simulink subsystem "snake_main_model"  (R2022a)
settings: Solver=VariableStepAuto  StartTime=0.0  StopTime=10.0  RelTol=1e-3
settings Model: DefaultTestHarness=snake_main_model_harness  Creator=andre  LastModifiedBy=andre

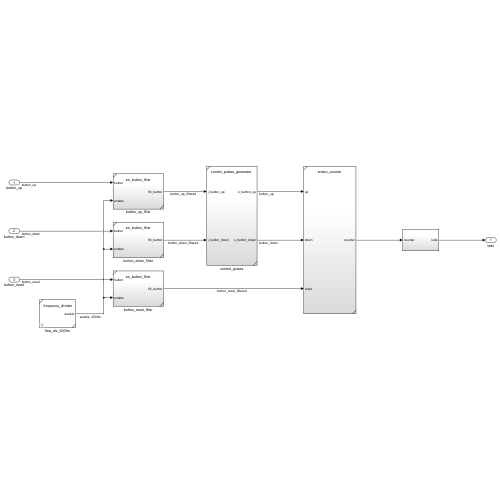
[thumbnail: Simulink's stored preview of the top-level diagram]
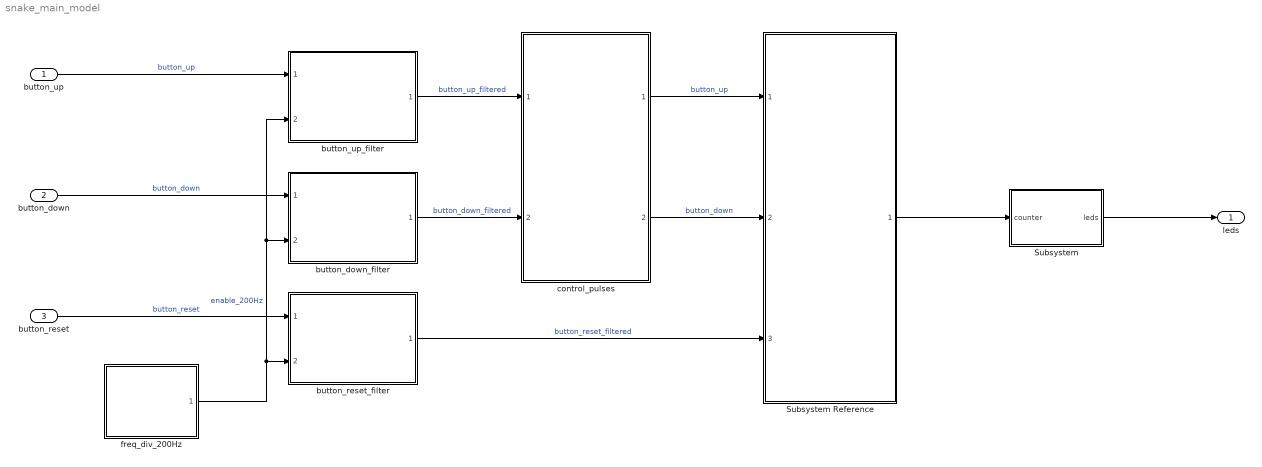
== system snake_main_model ==
  button_up : Inport  OutDataTypeStr=boolean  PortDimensions=1
  button_down : Inport  Port=2  OutDataTypeStr=boolean  PortDimensions=1
  button_reset : Inport  Port=3  OutDataTypeStr=boolean  PortDimensions=1
  Subsystem : Subsystem
  Subsystem Reference : Subsystem  ReferencedSubsystem=snake_counter
  button_down_filter : Subsystem  ReferencedSubsystem=en_button_filter
  button_reset_filter : Subsystem  ReferencedSubsystem=en_button_filter
  button_up_filter : Subsystem  ReferencedSubsystem=en_button_filter
  control_pulses : Subsystem  ReferencedSubsystem=control_pulses_generator
  freq_div_200Hz : Subsystem  ReferencedSubsystem=frequency_divider  N=1e6
  leds : Outport  OutDataTypeStr=boolean  PortDimensions=8
  wires:
  button_up/1 -> button_up_filter/1  "button_up"
  button_down/1 -> button_down_filter/1  "button_down"
  button_reset/1 -> button_reset_filter/1  "button_reset"
  freq_div_200Hz/1 -> button_up_filter/2, button_down_filter/2, button_reset_filter/2  "enable_200Hz"
  button_reset_filter/1 -> Subsystem Reference/3  "button_reset_filtered"
  button_up_filter/1 -> control_pulses/1  "button_up_filtered"
  button_down_filter/1 -> control_pulses/2  "button_down_filtered"
  control_pulses/1 -> Subsystem Reference/1  "button_up"
  control_pulses/2 -> Subsystem Reference/2  "button_down"
  Subsystem Reference/1 -> Subsystem/1(counter)
  Subsystem/1(leds) -> leds/1

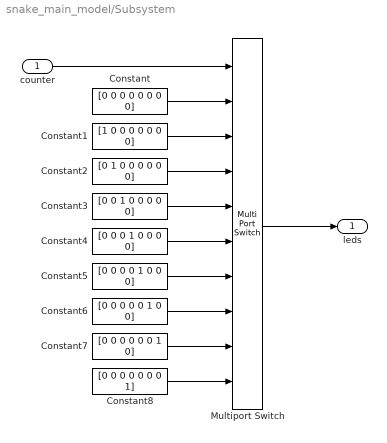
== system snake_main_model/Subsystem ==
  counter : Inport
  Constant : Constant  Value=[0 0 0 0 0 0 0 0]  OutDataTypeStr=boolean  SampleTime=-1
  Constant1 : Constant  Value=[1 0 0 0 0 0 0 0]  OutDataTypeStr=boolean  SampleTime=-1
  Constant2 : Constant  Value=[0 1 0 0 0 0 0 0]  OutDataTypeStr=boolean  SampleTime=-1
  Constant3 : Constant  Value=[0 0 1 0 0 0 0 0]  OutDataTypeStr=boolean  SampleTime=-1
  Constant4 : Constant  Value=[0 0 0 1 0 0 0 0]  OutDataTypeStr=boolean  SampleTime=-1
  Constant5 : Constant  Value=[0 0 0 0 1 0 0 0]  OutDataTypeStr=boolean  SampleTime=-1
  Constant6 : Constant  Value=[0 0 0 0 0 1 0 0]  OutDataTypeStr=boolean  SampleTime=-1
  Constant7 : Constant  Value=[0 0 0 0 0 0 1 0]  OutDataTypeStr=boolean  SampleTime=-1
  Constant8 : Constant  Value=[0 0 0 0 0 0 0 1]  OutDataTypeStr=boolean  SampleTime=-1
  Multiport Switch : MultiPortSwitch  DataPortOrder=Zero-based contiguous  Inputs=9  zeroidx=on  SaturateOnIntegerOverflow=off  InputSameDT=off
  leds : Outport
  wires:
  counter/1 -> Multiport Switch/1
  Multiport Switch/1 -> leds/1
  Constant/1 -> Multiport Switch/2
  Constant1/1 -> Multiport Switch/3
  Constant2/1 -> Multiport Switch/4
  Constant3/1 -> Multiport Switch/5
  Constant4/1 -> Multiport Switch/6
  Constant5/1 -> Multiport Switch/7
  Constant6/1 -> Multiport Switch/8
  Constant7/1 -> Multiport Switch/9
  Constant8/1 -> Multiport Switch/10
